simulink model "induction_motor_Vector_control_v1"  (R2017b)
settings: Solver=FixedStepAuto  StartTime=0.0  StopTime=1  FixedStep=0.0001  MaxStep=0.0001  RelTol=1e-3
values from neighbouring files (symbols this model uses):
  A1 = [-1/(Ts*sig) 0 M/(Ls*Tr*sig) 0; 0 -1/(Ts*sig) 0 M/(Ls*Tr*sig); M/(Lr*Ts*sig) 0 -1/(Tr*sig) 0 ; 0 M/(Ls*Ts*sig) 0 -1/(Tr*sig)]    [IM_vector_control_init.m]
  A2 = [0 1 0 0; -1 0 0 0 ; 0 0 0 1 ; 0 0 -1 0]    [IM_vector_control_init.m]
  A3 = [0 1/sig 0 M/(Ls*sig); -1/sig 0 -M/(Ls*sig) 0 ; 0 -M/(Lr*sig) 0 -M^2/(Ls*Lr*sig) ; M/(Lr*sig) 0 M^2/(Ls*Lr*sig) 0]    [IM_vector_control_init.m]
  B = [1/(Ls*sig) 0 0 0; 0 1/(Ls*sig) 0 0; -M/(Ls*Lr*sig) 0 0 0; 0 -M/(Ls*Lr*sig) 0 0 ]    [IM_vector_control_init.m]
  C = [Rs 0 0; 0 Rs 0]    [IM_vector_control_init.m]
  D = [0 -sig*Ls 0; sig*Ls 0 M/Lr]    [IM_vector_control_init.m]
  fpor = 5000    [IM_vector_control_init.m]
  fr = 0    [IM_vector_control_init.m]
  J = 0.031    [IM_vector_control_init.m]
  L = [Ls 0 M 0 ; 0 Ls 0 M; M 0 Lr 0; 0 M 0 Lr]    [IM_vector_control_init.m]
  Lr = 0.274    [IM_vector_control_init.m]
  M = 0.258    [IM_vector_control_init.m]
  p = 2    [IM_vector_control_init.m]
  T = [2/3 -1/3 -1/3;-1/3 2/3 -1/3;-1/3 -1/3 2/3]    [IM_vector_control_init.m]
  Tr = Lr/Rr    (= 0.0720105124836)    [IM_vector_control_init.m]
undefined symbols (not defined in the file or in its folder): f
libraries: simulink x3
settings Model: SimulationMode=accelerator  Creator=proso  LastModifiedBy=proso

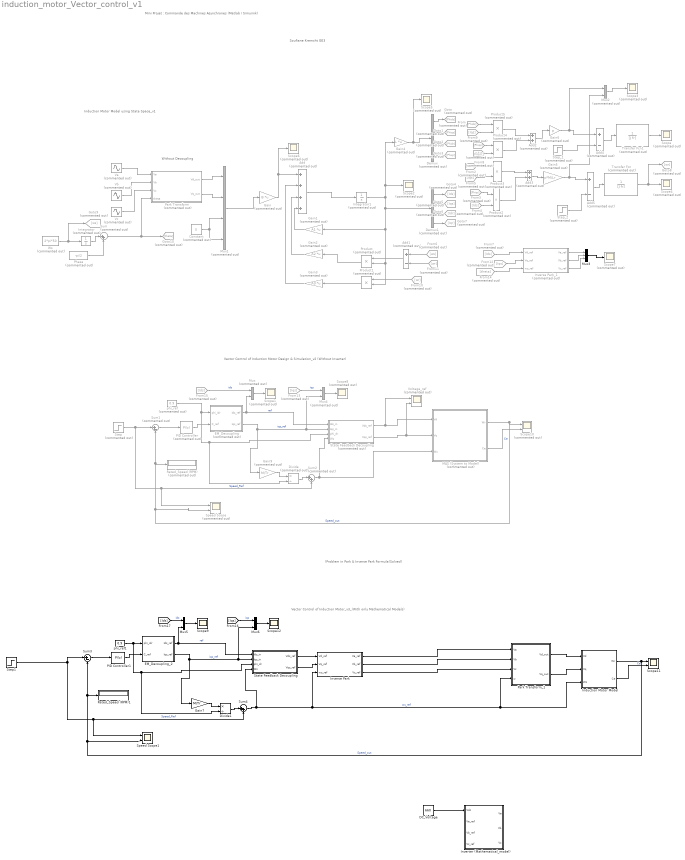
== system induction_motor_Vector_control_v1 ==
  note: (Problem in Park & Inverse Park Formula(Solved)
  note: Soufiane Kremcht GE3
  note: Without Decoupling
  note: Induction Motor Model using State Space_v1
  note: Vector Control of Induction Motor Design & Simulation_v2 (Without Inverter)
  note: Vector Control of Induction Motor_v3_(With only Mathematical Models)
  note: Mini Projet : Commande des Machines Asynchrones (Matlab / Simuiink)
  Add : Sum  Commented=on  Inputs=4
  Add1 : Sum  Commented=on  Inputs=+-
  Add2 : Sum  Commented=on
  Add3 : Sum  Commented=on
  Add4 : Sum  Commented=on  Inputs=+-
  Add5 : Sum  Commented=on  Inputs=+-
  Constant : Constant  Commented=on  Value=0
  DC_Voltage : Constant  Value=660
  Demux : Demux  Commented=on
  Demux1 : Demux  Commented=on
  Divide : Product  Commented=on  Inputs=*/
  Divide1 : Product  Inputs=*/
  EM_Decoupling : Subsystem  Commented=on
  EM_Decoupling_2 : Subsystem
  From : From  Commented=on  GotoTag=Phids
  From1 : From  Commented=on  GotoTag=Phiqs
  From10 : From  Commented=on  GotoTag=wr
  From11 : From  Commented=on  GotoTag=wr
  From{5,9,12..13} (4 alike) : From  Commented=on  GotoTag=Iqs
  From14 : From  Commented=on  GotoTag=theta
  From{4,7..8,15} (4 alike) : From  Commented=on  GotoTag=Ids
  From2 : From  Commented=on  GotoTag=Phidr
  From3 : From  Commented=on  GotoTag=Phiqr
  From6 : From  Commented=on  GotoTag=ws
  Gain : Gain  Commented=on  Gain=B  Multiplication=Matrix(K*u)
  Gain1 : Gain  Commented=on  Gain=A1  Multiplication=Matrix(K*u)
  Gain2 : Gain  Commented=on  Gain=A2  Multiplication=Matrix(K*u)
  Gain3 : Gain  Commented=on  Gain=A3  Multiplication=Matrix(K*u)
  Gain4 : Gain  Commented=on  Gain=L  Multiplication=Matrix(K*u)
  Gain5 : Gain  Commented=on  Gain=p*M/Lr
  Gain6 : Gain  Commented=on  Gain=p
  Gain7 : Gain  Gain=M/Tr
  Gain9 : Gain  Commented=on  Gain=M/Tr
  Goto : Goto  Commented=on  GotoTag=Phids
  Goto1 : Goto  Commented=on  GotoTag=Phiqs
  Goto10 : Goto  Commented=on  GotoTag=theta
  Goto2 : Goto  Commented=on  GotoTag=Phidr
  Goto3 : Goto  Commented=on  GotoTag=Phiqr
  Goto4 : Goto  Commented=on  GotoTag=Ids
  Goto5 : Goto  Commented=on  GotoTag=Iqs
  Goto6 : Goto  Commented=on  GotoTag=Idr
  Goto7 : Goto  Commented=on  GotoTag=Iqr
  Goto8 : Goto  Commented=on  GotoTag=wr
  Goto9 : Goto  Commented=on  GotoTag=ws
  Induction Motor Model : Subsystem
  Integrator : Integrator  Commented=on
  Integrator1 : Integrator  Commented=on
  Inverse Park : Subsystem
  Inverse Park_1 : Subsystem  Commented=on
  Inverter (Mathematical_model) : Subsystem
  MAS (System to Model) : Subsystem  Commented=on
  Mux : Mux  Commented=on  Inputs=2
  Mux1 : Mux  Commented=on
  Mux2 : Mux  Commented=on  Inputs=2
  Mux3 : Mux  Inputs=3
  Mux4 : Mux  Commented=on  Inputs=2
  Mux5 : Mux  Inputs=2
  Mux6 : Mux  Inputs=2
  PID Controller : simulink/Continuous/PID Controller  Commented=on  Controller=PI  TimeDomain=Discrete-time  SampleTime=-1  IntegratorMethod=Forward Euler  FilterMethod=Forward Euler  Form=Parallel  UseFilter=on  ControllerParametersSource=internal  P=1  I=1  D=1  N=100  InitialConditionSource=internal  InitialConditionForIntegrator=0  InitialConditionForFilter=0  ExternalReset=none  LimitOutput=off  UpperSaturationLimit=inf  LowerSaturationLimit=-inf  LinearizeAsGain=on  AntiWindupMode=none  Kb=1  TrackingMode=off  Kt=1  PParamMin=[]  PParamMax=[]  IParamMin=[]  IParamMax=[]  DParamMin=[]  DParamMax=[]  NParamMin=[]  NParamMax=[]  KbParamMin=[]  KbParamMax=[]  KtParamMin=[]  KtParamMax=[]  POutMin=[]  POutMax=[]  IOutMin=[]  IOutMax=[]  DOutMin=[]  DOutMax=[]  NOutMin=[]  NOutMax=[]  KbOutMin=[]  KbOutMax=[]  KtOutMin=[]  KtOutMax=[]  IntegratorOutMin=[]  IntegratorOutMax=[]  FilterOutMin=[]  FilterOutMax=[]  SumOutMin=[]  SumOutMax=[]  SumI1OutMin=[]  SumI1OutMax=[]  SumI2OutMin=[]  SumI2OutMax=[]  SumI3OutMin=[]  SumI3OutMax=[]  SumDOutMin=[]  SumDOutMax=[]  SaturationOutMin=[]  SaturationOutMax=[]  IntegratorContinuousStateAttributes=''  IntegratorStateMustResolveToSignalObject=off  IntegratorRTWStateStorageClass=Auto  FilterContinuousStateAttributes=''  FilterStateMustResolveToSignalObject=off  FilterRTWStateStorageClass=Auto  DifferentiatorICPrevScaledInput=0  DifferentiatorOutMin=[]  DifferentiatorOutMax=[]  InitialConditionSetting=State (most efficient)  FilterDiffOutCoefMin=[]  FilterDiffOutCoefMax=[]  SumDenOutMin=[]  SumDenOutMax=[]  SumNumOutMin=[]  SumNumOutMax=[]  ReciprocalOutMin=[]  ReciprocalOutMax=[]  DivideOutMin=[]  DivideOutMax=[]  TunerSelectOption=Transfer Function Based (PID Tuner App)
  PID Controller1 : simulink/Continuous/PID Controller  Controller=PI  TimeDomain=Discrete-time  SampleTime=-1  IntegratorMethod=Forward Euler  FilterMethod=Forward Euler  Form=Parallel  UseFilter=on  ControllerParametersSource=internal  P=1  I=2  D=1  N=100  InitialConditionSource=internal  InitialConditionForIntegrator=0  InitialConditionForFilter=0  ExternalReset=none  LimitOutput=off  UpperSaturationLimit=inf  LowerSaturationLimit=-inf  LinearizeAsGain=on  AntiWindupMode=none  Kb=1  TrackingMode=off  Kt=1  PParamMin=[]  PParamMax=[]  IParamMin=[]  IParamMax=[]  DParamMin=[]  DParamMax=[]  NParamMin=[]  NParamMax=[]  KbParamMin=[]  KbParamMax=[]  KtParamMin=[]  KtParamMax=[]  POutMin=[]  POutMax=[]  IOutMin=[]  IOutMax=[]  DOutMin=[]  DOutMax=[]  NOutMin=[]  NOutMax=[]  KbOutMin=[]  KbOutMax=[]  KtOutMin=[]  KtOutMax=[]  IntegratorOutMin=[]  IntegratorOutMax=[]  FilterOutMin=[]  FilterOutMax=[]  SumOutMin=[]  SumOutMax=[]  SumI1OutMin=[]  SumI1OutMax=[]  SumI2OutMin=[]  SumI2OutMax=[]  SumI3OutMin=[]  SumI3OutMax=[]  SumDOutMin=[]  SumDOutMax=[]  SaturationOutMin=[]  SaturationOutMax=[]  IntegratorContinuousStateAttributes=''  IntegratorStateMustResolveToSignalObject=off  IntegratorRTWStateStorageClass=Auto  FilterContinuousStateAttributes=''  FilterStateMustResolveToSignalObject=off  FilterRTWStateStorageClass=Auto  DifferentiatorICPrevScaledInput=0  DifferentiatorOutMin=[]  DifferentiatorOutMax=[]  InitialConditionSetting=State (most efficient)  FilterDiffOutCoefMin=[]  FilterDiffOutCoefMax=[]  SumDenOutMin=[]  SumDenOutMax=[]  SumNumOutMin=[]  SumNumOutMax=[]  ReciprocalOutMin=[]  ReciprocalOutMax=[]  DivideOutMin=[]  DivideOutMax=[]  TunerSelectOption=Transfer Function Based (PID Tuner App)
  Park Transform : Subsystem  Commented=on
  Park Transform_1 : Subsystem
  Phase : Constant  Commented=on  Value=-pi/2
  Product{,1..5} (6 alike) : Product  Commented=on
  Rated_Speed (RPM) : Display  Commented=on
  Rated_Speed (RPM)1 : Display
  Scope{,1..8} (9 alike) : Scope  Commented=on
  Scope10 : Scope  Commented=on  NumInputPorts=2
  Scope11 : Scope  NumInputPorts=2
  Scope12 : Scope
  Scope9 : Scope
  Speed Scope : Scope  Commented=on  NumInputPorts=2
  Speed Scope1 : Scope  NumInputPorts=2
  State Feedback Decoupling : Subsystem  Commented=on
  "State Feedback Decoupling " : Subsystem
  Step : Step  Commented=on  Time=4  Before=500  After=1000  SampleTime=0
  Step1 : Step  Time=0.5  Before=500  After=1000  SampleTime=0
  Step_1 : Step  Commented=on  Before=2  After=2  SampleTime=0
  Step_2 : Step  Commented=on  Before=2  After=2  SampleTime=0
  Sum : Sum  Commented=on  Inputs=|++
  Sum1 : Sum  Commented=on  Inputs=|+-
  Sum2 : Sum  Commented=on  Inputs=|++
  Sum3 : Sum  Inputs=|+-
  Sum4 : Sum  Inputs=|++
  Transfer Fcn : TransferFcn  Commented=on  Denominator=[J fr]
  Transfer Fcn1 : TransferFcn  Commented=on  Denominator=[J fr]
  Va : Sin  Commented=on  Amplitude=240  Frequency=2*pi*f  SampleTime=0
  Vb : Sin  Commented=on  Amplitude=240  Frequency=2*pi*f  Phase=-2*pi/3  SampleTime=0
  Vc : Sin  Commented=on  Amplitude=240  Frequency=2*pi*f  Phase=2*pi/3  SampleTime=0
  Voltage_ref : Scope  Commented=on  NumInputPorts=2
  Ws : Constant  Commented=on  Value=2*pi*50
  phi_ref : Constant  Commented=on  Value=0.9
  phi_ref1 : Constant  Value=0.9
  wires:
  Integrator/1 -> Sum/1
  Ws/1 -> Goto9/1, Integrator/1
  Phase/1 -> Sum/2
  Integrator1/1 -> Gain1/1, Product/2, Product1/2, Demux1/1, Scope2/1, Gain4/1
  Add/1 -> Integrator1/1
  Constant/1 -> Mux1/4, Mux1/3
  Mux1/1 -> Gain/1
  Gain/1 -> Add/1, Scope6/1
  Gain4/1 -> Scope5/1, Demux/1
  Product/1 -> Gain2/1
  Gain3/1 -> Add/2
  Gain2/1 -> Add/3
  Gain1/1 -> Add/4
  Mux2/1 -> Scope3/1
  Product5/1 -> Add2/1
  Product4/1 -> Add2/2
  Product3/1 -> Add3/1
  Product2/1 -> Add3/2
  Demux/1 -> Goto/1
  Step_1/1 -> Add4/2
  Add2/1 -> Gain6/1
  Gain6/1 -> Mux2/1, Add4/1
  Transfer Fcn/1 -> Goto8/1, Scope4/1
  Add5/1 -> Transfer Fcn/1
  Add3/1 -> Gain5/1
  Gain5/1 -> Mux2/2, Add5/1
  Step_2/1 -> Add5/2
  Add1/1 -> Product/1
  Product1/1 -> Gain3/1
  Demux/2 -> Goto1/1
  Demux/3 -> Goto2/1
  Demux/4 -> Goto3/1
  Demux1/1 -> Goto4/1
  Demux1/2 -> Goto5/1
  Demux1/3 -> Goto6/1
  Demux1/4 -> Goto7/1
  From4/1 -> Product2/2
  From3/1 -> Product2/1
  From8/1 -> Product4/2
  From/1 -> Product5/1
  From1/1 -> Product4/1
  From5/1 -> Product3/2
  From9/1 -> Product5/2
  From2/1 -> Product3/1
  Add4/1 -> Transfer Fcn1/1
  Transfer Fcn1/1 -> Scope/1
  From10/1 -> Product1/1
  From11/1 -> Add1/2
  From6/1 -> Add1/1
  From7/1 -> Inverse Park_1/1(Vd_ref)
  From12/1 -> Inverse Park_1/2(Vq_ref)
  From14/1 -> Inverse Park_1/3(ws_ref)
  Mux3/1 -> Scope7/1
  Va/1 -> Park Transform/1(Va)
  Vb/1 -> Park Transform/2(Vb)
  Vc/1 -> Park Transform/3(Vc)
  Sum/1 -> Park Transform/4(theta), Goto10/1
  Park Transform/1(Vd_out) -> Mux1/1
  Park Transform/2(Vq_out) -> Mux1/2
  MAS (System to Model)/1(Wr) -> Speed Scope/2, Rated_Speed (RPM)/1, Sum1/2, Scope10/1  "Speed_out"
  MAS (System to Model)/2(Ce) -> Scope10/2  "Ce"
  Sum1/1 -> PID Controller/1
  Step/1 -> Sum1/1, Speed Scope/1, Sum2/2  "Speed_Ref"
  PID Controller/1 -> EM_Decoupling/2(C_ref)
  phi_ref/1 -> State Feedback Decoupling/3(phi_dr), Divide/2, EM_Decoupling/1(phi_idr)
  EM_Decoupling/2(Iqs_ref) -> Mux4/2, State Feedback Decoupling/2(Iqs_in), Gain9/1  "iqs_ref"
  Gain9/1 -> Divide/1
  Divide/1 -> Sum2/1
  EM_Decoupling/1(Ids_ref) -> Mux/2, State Feedback Decoupling/1(Ids_in)  "ref"
  Sum2/1 -> MAS (System to Model)/3(Ws), State Feedback Decoupling/4(Ws)
  State Feedback Decoupling/1(Vds_ref) -> Voltage_ref/1, MAS (System to Model)/1(Vd)
  State Feedback Decoupling/2(Vqs_ref) -> Voltage_ref/2, MAS (System to Model)/2(Vq)
  From15/1 -> Mux/1  "ids"
  Mux/1 -> Scope1/1
  Mux4/1 -> Scope8/1
  From13/1 -> Mux4/1  "iqs"
  Sum3/1 -> PID Controller1/1
  Mux6/1 -> Scope12/1
  [Ids] -> Mux5/1  "ids"
  Step1/1 -> Sum3/1, Speed Scope1/1, Sum4/2  "Speed_Ref"
  PID Controller1/1 -> EM_Decoupling_2/2(C_ref)
  Mux5/1 -> Scope9/1
  Gain7/1 -> Divide1/1
  EM_Decoupling_2/2(Iqs_ref) -> Mux6/2, "State Feedback Decoupling "/2(Iqs_in), Gain7/1  "iqs_ref"
  Divide1/1 -> Sum4/1
  Sum4/1 -> Park Transform_1/4(w), Induction Motor Model/3(Ws), Inverse Park/3(ws_ref), "State Feedback Decoupling "/4(Ws)  "ws_ref"
  [Iqs] -> Mux6/1  "iqs"
  EM_Decoupling_2/1(Ids_ref) -> Mux5/2, "State Feedback Decoupling "/1(Ids_in)  "ref"
  phi_ref1/1 -> "State Feedback Decoupling "/3(phi_dr), Divide1/2, EM_Decoupling_2/1(phi_idr)
  Induction Motor Model/2(Ce) -> Scope11/2  "Ce"
  Induction Motor Model/1(Wr) -> Scope11/1, Speed Scope1/2, Rated_Speed (RPM)1/1, Sum3/2  "Speed_out"
  "State Feedback Decoupling "/2(Vqs_ref) -> Inverse Park/2(Vq_ref)
  "State Feedback Decoupling "/1(Vds_ref) -> Inverse Park/1(Vd_ref)
  Park Transform_1/1(Vd_out) -> Induction Motor Model/1(Vd)
  Park Transform_1/2(Vq_out) -> Induction Motor Model/2(Vq)
  Inverse Park_1/1(Va_ref) -> Mux3/1
  Inverse Park_1/2(Vb_ref) -> Mux3/2
  Inverse Park_1/3(Vc_ref) -> Mux3/3
  Inverse Park/1(Va_ref) -> Park Transform_1/1(Va)
  Inverse Park/2(Vb_ref) -> Park Transform_1/2(Vb)
  Inverse Park/3(Vc_ref) -> Park Transform_1/3(Vc)
  DC_Voltage/1 -> Inverter (Mathematical_model)/1(Vdc)

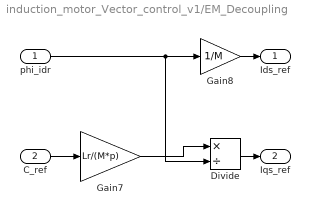
== system induction_motor_Vector_control_v1/EM_Decoupling ==
  phi_idr : Inport
  C_ref : Inport  Port=2
  Divide : Product  Inputs=*/
  Gain7 : Gain  Gain=Lr/(M*p)
  Gain8 : Gain  Gain=1/M
  Ids_ref : Outport
  Iqs_ref : Outport  Port=2
  wires:
  Gain8/1 -> Ids_ref/1
  Divide/1 -> Iqs_ref/1
  C_ref/1 -> Gain7/1
  Gain7/1 -> Divide/1
  phi_idr/1 -> Divide/2, Gain8/1

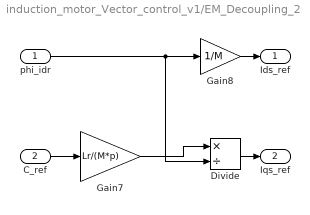
== system induction_motor_Vector_control_v1/EM_Decoupling_2 ==
  phi_idr : Inport
  C_ref : Inport  Port=2
  Divide : Product  Inputs=*/
  Gain7 : Gain  Gain=Lr/(M*p)
  Gain8 : Gain  Gain=1/M
  Ids_ref : Outport
  Iqs_ref : Outport  Port=2
  wires:
  Gain8/1 -> Ids_ref/1
  Divide/1 -> Iqs_ref/1
  C_ref/1 -> Gain7/1
  Gain7/1 -> Divide/1
  phi_idr/1 -> Divide/2, Gain8/1

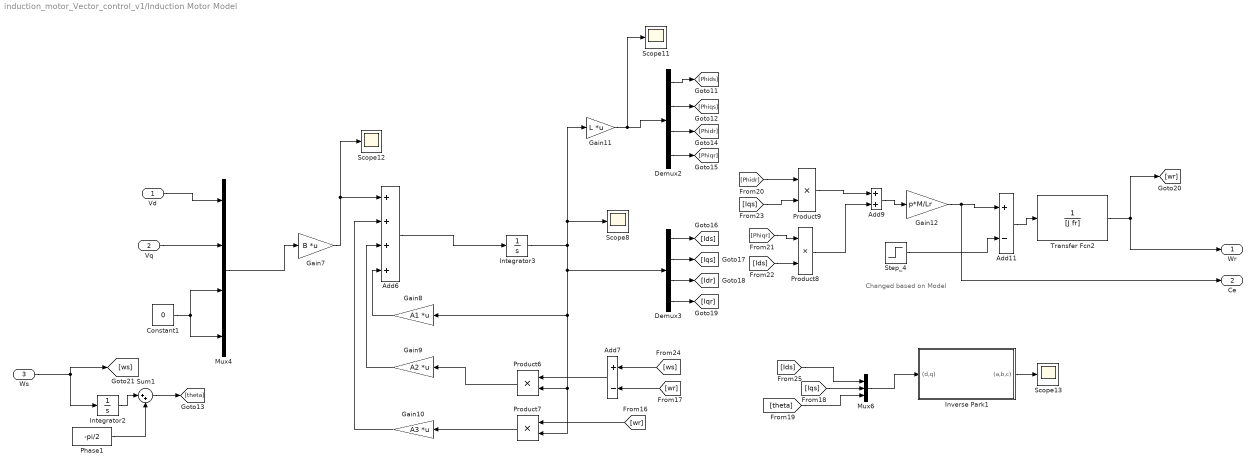
== system induction_motor_Vector_control_v1/Induction Motor Model ==
  note: Changed based on Model
  Vd : Inport
  Vq : Inport  Port=2
  Ws : Inport  Port=3
  Add11 : Sum  Inputs=+-
  Add6 : Sum  Inputs=4
  Add7 : Sum  Inputs=+-
  Add9 : Sum
  Constant1 : Constant  Value=0
  Demux2 : Demux
  Demux3 : Demux
  Gain10 : Gain  Gain=A3  Multiplication=Matrix(K*u)
  Gain11 : Gain  Gain=L  Multiplication=Matrix(K*u)
  Gain12 : Gain  Gain=p*M/Lr
  Gain7 : Gain  Gain=B  Multiplication=Matrix(K*u)
  Gain8 : Gain  Gain=A1  Multiplication=Matrix(K*u)
  Gain9 : Gain  Gain=A2  Multiplication=Matrix(K*u)
  Integrator2 : Integrator
  Integrator3 : Integrator
  Inverse Park1 : Subsystem
  Mux4 : Mux
  Mux6 : Mux  Inputs=3
  Phase1 : Constant  Value=-pi/2
  Product{6..9} (4 alike) : Product
  Scope{8,11..13} (4 alike) : Scope
  Step_4 : Step  Time=5  Before=0.5  After=10  SampleTime=0
  Sum1 : Sum  Inputs=|++
  Transfer Fcn2 : TransferFcn  Denominator=[J fr]
  Wr : Outport
  Ce : Outport  Port=2
  wires:
  Gain9/1 -> Add6/3
  Inverse Park1/1((a,b,c)) -> Scope13/1
  Demux3/2 -> [Iqs]
  Demux3/3 -> [Idr]
  Integrator3/1 -> Gain8/1, Product6/2, Product7/2, Demux3/1, Scope8/1, Gain11/1
  Demux2/4 -> [Phiqr]
  Gain12/1 -> Ce/1, Add11/1
  [theta] -> Mux6/3
  [wr] -> Product7/1
  [Iqs] -> Product9/2
  Add9/1 -> Gain12/1
  [Iqs] -> Mux6/2
  Vd/1 -> Mux4/1
  Ws/1 -> Integrator2/1, [ws]
  Demux2/2 -> [Phiqs]
  Add11/1 -> Transfer Fcn2/1
  Demux2/1 -> [Phids]
  Gain11/1 -> Scope11/1, Demux2/1
  Product7/1 -> Gain10/1
  [Ids] -> Mux6/1
  Sum1/1 -> [theta]
  Vq/1 -> Mux4/2
  Product8/1 -> Add9/2
  [Phidr] -> Product9/1
  Add7/1 -> Product6/1
  Constant1/1 -> Mux4/4, Mux4/3
  Mux4/1 -> Gain7/1
  [ws] -> Add7/1
  Demux2/3 -> [Phidr]
  Demux3/4 -> [Iqr]
  Integrator2/1 -> Sum1/1
  Gain8/1 -> Add6/4
  Add6/1 -> Integrator3/1
  Product9/1 -> Add9/1
  [wr] -> Add7/2
  Product6/1 -> Gain9/1
  Gain7/1 -> Add6/1, Scope12/1
  Transfer Fcn2/1 -> Wr/1, [wr]
  Mux6/1 -> Inverse Park1/1((d,q))
  Demux3/1 -> [Ids]
  Phase1/1 -> Sum1/2
  Step_4/1 -> Add11/2
  [Phiqr] -> Product8/1
  [Ids] -> Product8/2
  Gain10/1 -> Add6/2

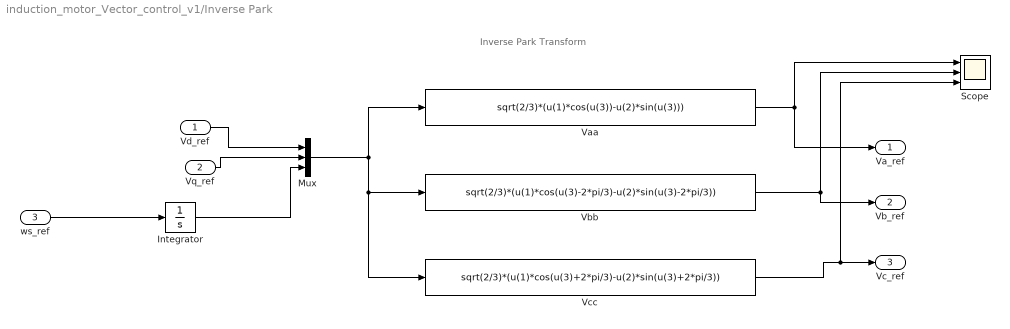
== system induction_motor_Vector_control_v1/Inverse Park ==
  note: Inverse Park Transform
  Vd_ref : Inport
  Vq_ref : Inport  Port=2
  ws_ref : Inport  Port=3
  Integrator : Integrator
  Mux : Mux  Inputs=3
  Scope : Scope  NumInputPorts=3
  Vaa : Fcn  Expr=sqrt(2/3)*(u(1)*cos(u(3))-u(2)*sin(u(3)))
  Vbb : Fcn  Expr=sqrt(2/3)*(u(1)*cos(u(3)-2*pi/3)-u(2)*sin(u(3)-2*pi/3))
  Vcc : Fcn  Expr=sqrt(2/3)*(u(1)*cos(u(3)+2*pi/3)-u(2)*sin(u(3)+2*pi/3))
  Va_ref : Outport
  Vb_ref : Outport  Port=2
  Vc_ref : Outport  Port=3
  wires:
  Vd_ref/1 -> Mux/1
  Vq_ref/1 -> Mux/2
  ws_ref/1 -> Integrator/1
  Mux/1 -> Vcc/1, Vbb/1, Vaa/1
  Vaa/1 -> Va_ref/1, Scope/1
  Vbb/1 -> Vb_ref/1, Scope/2
  Vcc/1 -> Scope/3, Vc_ref/1
  Integrator/1 -> Mux/3

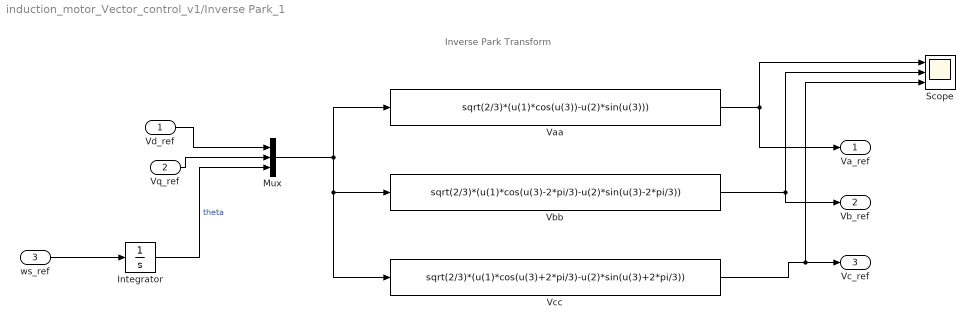
== system induction_motor_Vector_control_v1/Inverse Park_1 ==
  note: Inverse Park Transform
  Vd_ref : Inport
  Vq_ref : Inport  Port=2
  ws_ref : Inport  Port=3
  Integrator : Integrator
  Mux : Mux  Inputs=3
  Scope : Scope  NumInputPorts=3
  Vaa : Fcn  Expr=sqrt(2/3)*(u(1)*cos(u(3))-u(2)*sin(u(3)))
  Vbb : Fcn  Expr=sqrt(2/3)*(u(1)*cos(u(3)-2*pi/3)-u(2)*sin(u(3)-2*pi/3))
  Vcc : Fcn  Expr=sqrt(2/3)*(u(1)*cos(u(3)+2*pi/3)-u(2)*sin(u(3)+2*pi/3))
  Va_ref : Outport
  Vb_ref : Outport  Port=2
  Vc_ref : Outport  Port=3
  wires:
  Vd_ref/1 -> Mux/1
  Vq_ref/1 -> Mux/2
  ws_ref/1 -> Integrator/1
  Mux/1 -> Vcc/1, Vbb/1, Vaa/1
  Vaa/1 -> Va_ref/1, Scope/1
  Vbb/1 -> Vb_ref/1, Scope/2
  Vcc/1 -> Scope/3, Vc_ref/1
  Integrator/1 -> Mux/3  "theta"

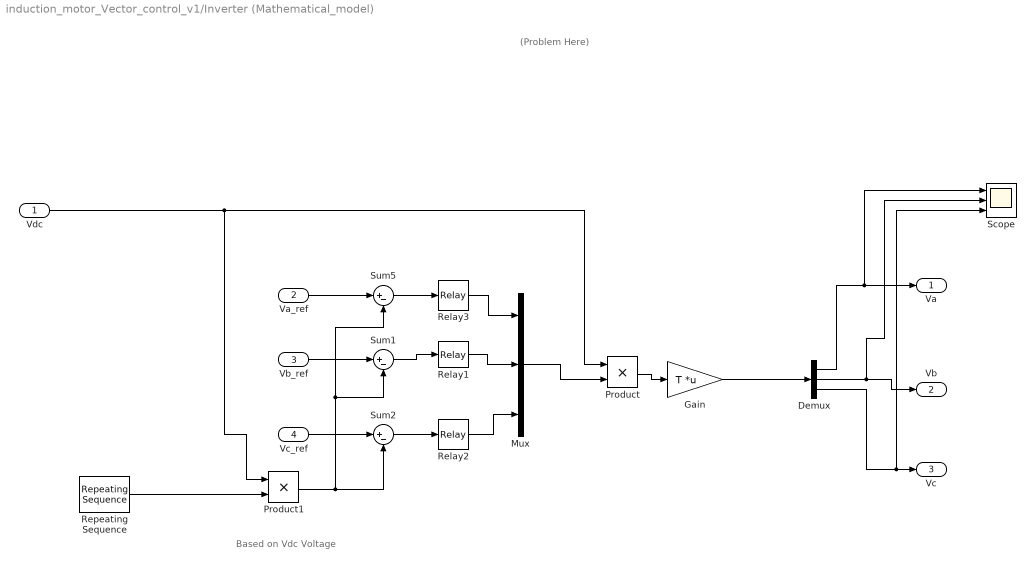
== system induction_motor_Vector_control_v1/Inverter (Mathematical_model) ==
  note: Based on Vdc Voltage
  note: (Problem Here)
  Vdc : Inport
  Va_ref : Inport  Port=2
  Vb_ref : Inport  Port=3
  Vc_ref : Inport  Port=4
  Demux : Demux  Outputs=3
  Gain : Gain  Gain=T  Multiplication=Matrix(K*u)
  Mux : Mux  Inputs=3
  Product : Product
  Product1 : Product
  Relay1 : Relay  OffOutputValue=-1
  Relay2 : Relay  OffOutputValue=-1
  Relay3 : Relay  OffOutputValue=-1
  Repeating Sequence : simulink/Sources/Repeating Sequence  rep_seq_t=[0 1/(2*fpor) 1/fpor]  rep_seq_y=[-1 1 -1]
  Scope : Scope  NumInputPorts=3
  Sum1 : Sum  Inputs=|+-
  Sum2 : Sum  Inputs=|+-
  Sum5 : Sum  Inputs=|+-
  Va : Outport
  Vb : Outport  Port=2
  Vc : Outport  Port=3
  wires:
  Sum5/1 -> Relay3/1
  Va_ref/1 -> Sum5/1
  Relay3/1 -> Mux/1
  Relay1/1 -> Mux/2
  Relay2/1 -> Mux/3
  Repeating Sequence/1 -> Product1/2
  Sum2/1 -> Relay2/1
  Sum1/1 -> Relay1/1
  Vb_ref/1 -> Sum1/1
  Product/1 -> Gain/1
  Mux/1 -> Product/2
  Vc_ref/1 -> Sum2/1
  Product1/1 -> Sum1/2, Sum5/2, Sum2/2
  Demux/1 -> Scope/1, Va/1
  Demux/2 -> Scope/2, Vb/1
  Demux/3 -> Scope/3, Vc/1
  Gain/1 -> Demux/1
  Vdc/1 -> Product1/1, Product/1

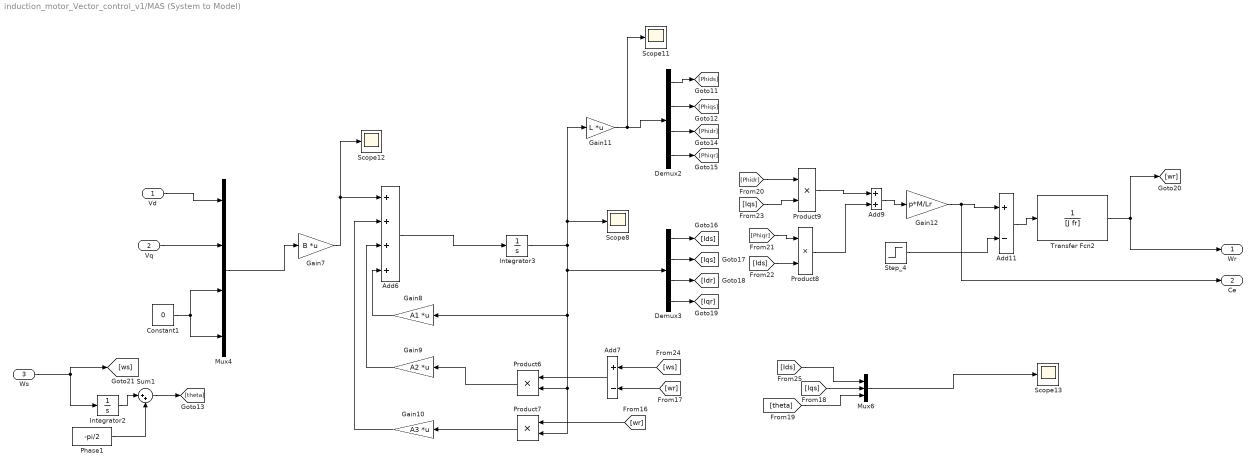
== system induction_motor_Vector_control_v1/MAS (System to Model) ==
  Vd : Inport
  Vq : Inport  Port=2
  Ws : Inport  Port=3
  Add11 : Sum  Inputs=+-
  Add6 : Sum  Inputs=4
  Add7 : Sum  Inputs=+-
  Add9 : Sum
  Constant1 : Constant  Value=0
  Demux2 : Demux
  Demux3 : Demux
  Gain10 : Gain  Gain=A3  Multiplication=Matrix(K*u)
  Gain11 : Gain  Gain=L  Multiplication=Matrix(K*u)
  Gain12 : Gain  Gain=p*M/Lr
  Gain7 : Gain  Gain=B  Multiplication=Matrix(K*u)
  Gain8 : Gain  Gain=A1  Multiplication=Matrix(K*u)
  Gain9 : Gain  Gain=A2  Multiplication=Matrix(K*u)
  Integrator2 : Integrator
  Integrator3 : Integrator
  Mux4 : Mux
  Mux6 : Mux  Inputs=3
  Phase1 : Constant  Value=-pi/2
  Product{6..9} (4 alike) : Product
  Scope{8,11..13} (4 alike) : Scope
  Step_4 : Step  Time=0.5  Before=0.5  SampleTime=0
  Sum1 : Sum  Inputs=|++
  Transfer Fcn2 : TransferFcn  Denominator=[J fr]
  Wr : Outport
  Ce : Outport  Port=2
  wires:
  Gain9/1 -> Add6/3
  Mux6/1 -> Scope13/1
  Demux3/2 -> [Iqs]
  Demux3/3 -> [Idr]
  Integrator3/1 -> Gain8/1, Product6/2, Product7/2, Demux3/1, Scope8/1, Gain11/1
  Demux2/4 -> [Phiqr]
  Gain12/1 -> Ce/1, Add11/1
  [theta] -> Mux6/3
  [wr] -> Product7/1
  [Iqs] -> Product9/2
  Add9/1 -> Gain12/1
  [Iqs] -> Mux6/2
  Vd/1 -> Mux4/1
  Ws/1 -> Integrator2/1, [ws]
  Demux2/2 -> [Phiqs]
  Add11/1 -> Transfer Fcn2/1
  Demux2/1 -> [Phids]
  Gain11/1 -> Scope11/1, Demux2/1
  Product7/1 -> Gain10/1
  [Ids] -> Mux6/1
  Sum1/1 -> [theta]
  Vq/1 -> Mux4/2
  Product8/1 -> Add9/2
  [Phidr] -> Product9/1
  Add7/1 -> Product6/1
  Constant1/1 -> Mux4/4, Mux4/3
  Mux4/1 -> Gain7/1
  [ws] -> Add7/1
  Demux2/3 -> [Phidr]
  Demux3/4 -> [Iqr]
  Integrator2/1 -> Sum1/1
  Gain8/1 -> Add6/4
  Add6/1 -> Integrator3/1
  Product9/1 -> Add9/1
  [wr] -> Add7/2
  Product6/1 -> Gain9/1
  Gain7/1 -> Add6/1, Scope12/1
  Transfer Fcn2/1 -> Wr/1, [wr]
  Demux3/1 -> [Ids]
  Phase1/1 -> Sum1/2
  Step_4/1 -> Add11/2
  [Phiqr] -> Product8/1
  [Ids] -> Product8/2
  Gain10/1 -> Add6/2

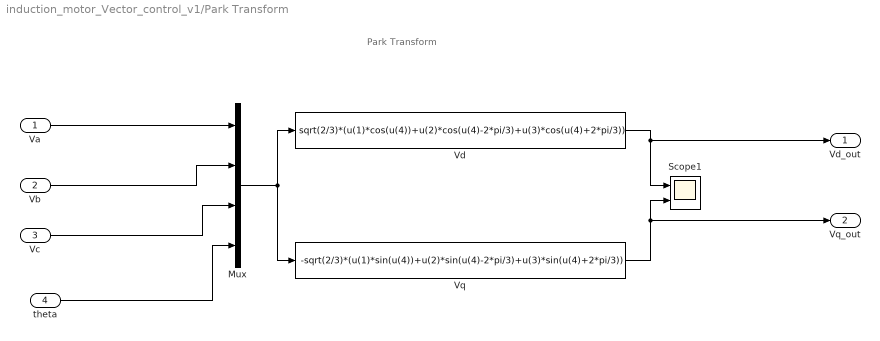
== system induction_motor_Vector_control_v1/Park Transform ==
  note: Park Transform
  Va : Inport
  Vb : Inport  Port=2
  Vc : Inport  Port=3
  theta : Inport  Port=4
  Mux : Mux
  Scope1 : Scope  NumInputPorts=2
  Vd : Fcn  Expr=sqrt(2/3)*(u(1)*cos(u(4))+u(2)*cos(u(4)-2*pi/3)+u(3)*cos(u(4)+2*pi/3))
  Vq : Fcn  Expr=-sqrt(2/3)*(u(1)*sin(u(4))+u(2)*sin(u(4)-2*pi/3)+u(3)*sin(u(4)+2*pi/3))
  Vd_out : Outport
  Vq_out : Outport  Port=2
  wires:
  Vb/1 -> Mux/2
  Va/1 -> Mux/1
  Vc/1 -> Mux/3
  Mux/1 -> Vq/1, Vd/1
  Vd/1 -> Vd_out/1, Scope1/1
  theta/1 -> Mux/4
  Vq/1 -> Vq_out/1, Scope1/2

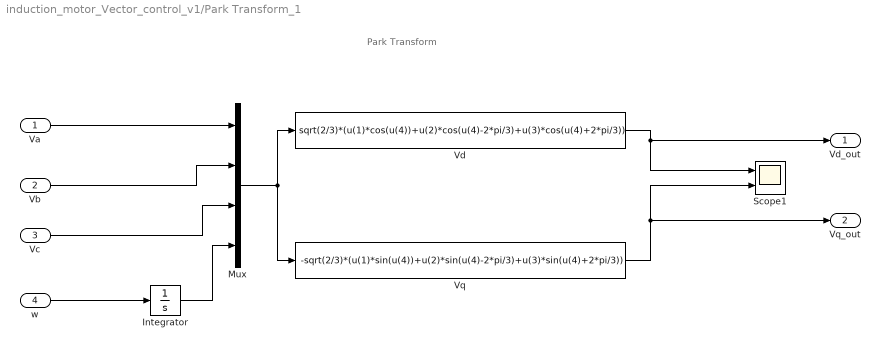
== system induction_motor_Vector_control_v1/Park Transform_1 ==
  note: Park Transform
  Va : Inport
  Vb : Inport  Port=2
  Vc : Inport  Port=3
  w : Inport  Port=4
  Integrator : Integrator
  Mux : Mux
  Scope1 : Scope  NumInputPorts=2
  Vd : Fcn  Expr=sqrt(2/3)*(u(1)*cos(u(4))+u(2)*cos(u(4)-2*pi/3)+u(3)*cos(u(4)+2*pi/3))
  Vq : Fcn  Expr=-sqrt(2/3)*(u(1)*sin(u(4))+u(2)*sin(u(4)-2*pi/3)+u(3)*sin(u(4)+2*pi/3))
  Vd_out : Outport
  Vq_out : Outport  Port=2
  wires:
  Vb/1 -> Mux/2
  Va/1 -> Mux/1
  Vc/1 -> Mux/3
  Mux/1 -> Vq/1, Vd/1
  Vd/1 -> Vd_out/1, Scope1/1
  w/1 -> Integrator/1
  Vq/1 -> Vq_out/1, Scope1/2
  Integrator/1 -> Mux/4

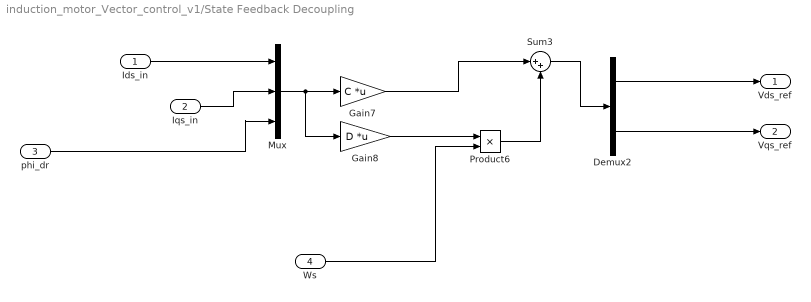
== system induction_motor_Vector_control_v1/State Feedback Decoupling ==
  Ids_in : Inport
  Iqs_in : Inport  Port=2
  phi_dr : Inport  Port=3
  Ws : Inport  Port=4
  Demux2 : Demux  Outputs=2
  Gain7 : Gain  Gain=C  Multiplication=Matrix(K*u)
  Gain8 : Gain  Gain=D  Multiplication=Matrix(K*u)
  Mux : Mux  Inputs=3
  Product6 : Product
  Sum3 : Sum  Inputs=|++
  Vds_ref : Outport
  Vqs_ref : Outport  Port=2
  wires:
  Iqs_in/1 -> Mux/2
  phi_dr/1 -> Mux/3
  Ids_in/1 -> Mux/1
  Mux/1 -> Gain8/1, Gain7/1
  Ws/1 -> Product6/2
  Gain8/1 -> Product6/1
  Sum3/1 -> Demux2/1
  Demux2/2 -> Vqs_ref/1
  Demux2/1 -> Vds_ref/1
  Gain7/1 -> Sum3/1
  Product6/1 -> Sum3/2

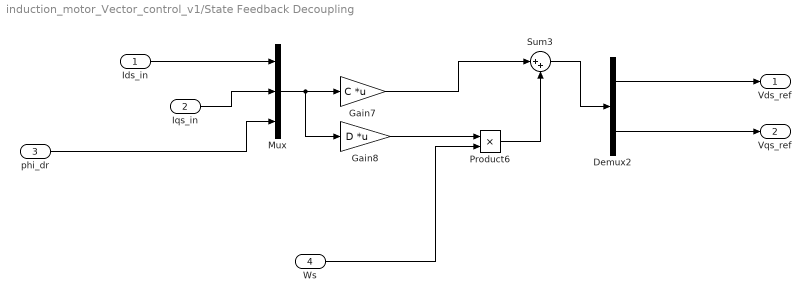
== system induction_motor_Vector_control_v1/State Feedback Decoupling  ==
  Ids_in : Inport
  Iqs_in : Inport  Port=2
  phi_dr : Inport  Port=3
  Ws : Inport  Port=4
  Demux2 : Demux  Outputs=2
  Gain7 : Gain  Gain=C  Multiplication=Matrix(K*u)
  Gain8 : Gain  Gain=D  Multiplication=Matrix(K*u)
  Mux : Mux  Inputs=3
  Product6 : Product
  Sum3 : Sum  Inputs=|++
  Vds_ref : Outport
  Vqs_ref : Outport  Port=2
  wires:
  Iqs_in/1 -> Mux/2
  phi_dr/1 -> Mux/3
  Ids_in/1 -> Mux/1
  Mux/1 -> Gain8/1, Gain7/1
  Ws/1 -> Product6/2
  Gain8/1 -> Product6/1
  Sum3/1 -> Demux2/1
  Demux2/2 -> Vqs_ref/1
  Demux2/1 -> Vds_ref/1
  Gain7/1 -> Sum3/1
  Product6/1 -> Sum3/2

== system induction_motor_Vector_control_v1/Induction Motor Model/Inverse Park1 ==
  note: Inverse Park Transform
  (d,q) : Inport
  Mux3 : Mux  Inputs=3
  Vaa : Fcn  Commented=on  Expr=sqrt(2/3)*(u(1)*cos(u(3))-u(2)*sin(u(3)))
  Vbb : Fcn  Commented=on  Expr=sqrt(2/3)*(u(1)*cos(u(3)-2*pi/3)-u(2)*sin(u(3)-2*pi/3))
  Vcc : Fcn  Commented=on  Expr=sqrt(2/3)*(u(1)*cos(u(3)+2*pi/3)-u(2)*sin(u(3)+2*pi/3))
  (a,b,c) : Outport
  wires:
  Vbb/1 -> Mux3/2
  (d,q)/1 -> Vaa/1, Vbb/1, Vcc/1
  Vaa/1 -> Mux3/1
  Vcc/1 -> Mux3/3
  Mux3/1 -> (a,b,c)/1
